simulink model "IM_DTC_controller_sim"  (R2023a)
settings: Solver=ode113  StartTime=0.0  StopTime=100.0  RelTol=1e-3
values from neighbouring files (symbols this model uses):
  B = 0.068    [IM_DTC_controller_param.m]
  DT = 0.001    [IM_DTC_controller_param.m]
  f = 50    [IM_DTC_controller_param.m]
  J = 0.4    [IM_DTC_controller_param.m]
  k = 0.009    [IM_DTC_controller_param.m]
  kiw = 0.068*1000    (= 68)    [IM_DTC_controller_param.m]
  kpw = 0.4*1000    (= 400)    [IM_DTC_controller_param.m]
  Lks = Ls- Lm^2/Lr    (= 0.00442538071066)    [IM_DTC_controller_param.m]
  Lm = 57e-3    (= 0.057)    [IM_DTC_controller_param.m]
  np = 3    [IM_DTC_controller_param.m]
  r = 4    [IM_DTC_controller_param.m]
  Rr = 0.175    [IM_DTC_controller_param.m]
  Rs = 0.24    [IM_DTC_controller_param.m]
  Rw = wc_des_w*(B+J*s)/s    [IM_DTC_controller_param.m]
  vsat = 380    [IM_DTC_controller_param.m]
  Ys_n = 1.71    [IM_DTC_controller_param.m]
undefined symbols (not defined in the file or in its folder): j
libraries: eeTransforms x5, sharedTrackingLibrary x1, slpidlib x1
settings Model: Creator=Andrea  LastModifiedBy=Andrea
settings SolverCC: ZeroCrossAlgorithm=Adaptive

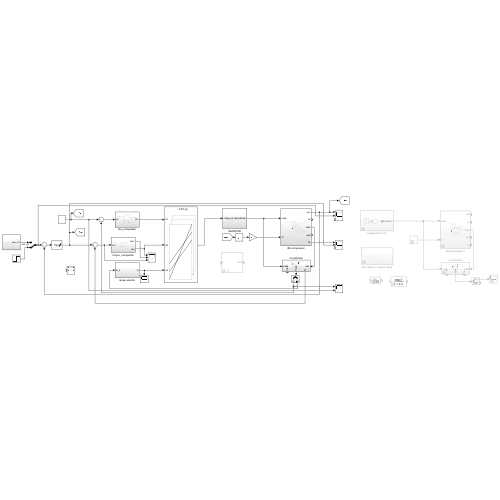
[thumbnail: Simulink's stored preview of the top-level diagram]
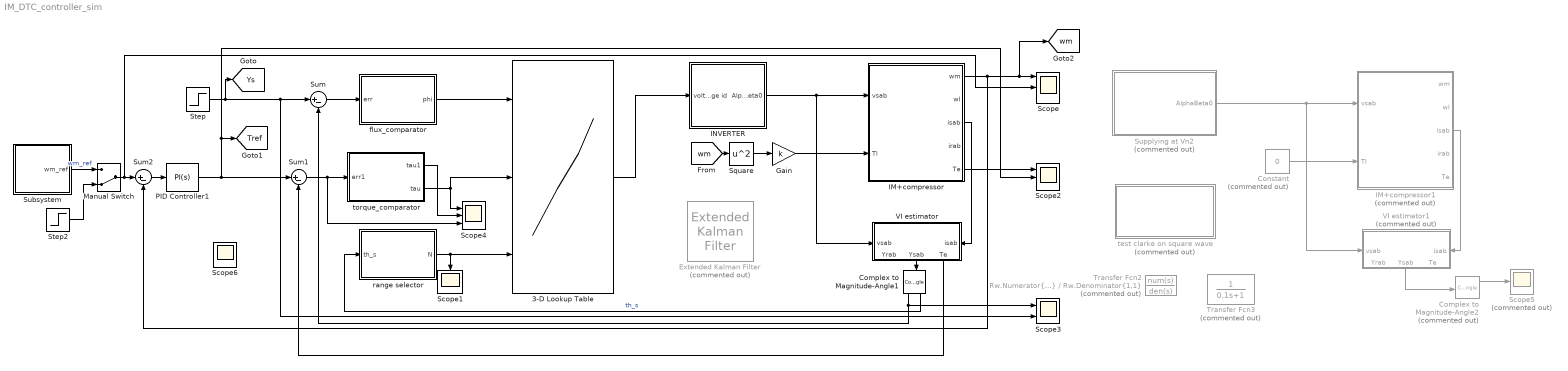
== system IM_DTC_controller_sim ==
  3-D Lookup Table : Lookup_n-D  NumberOfTableDimensions=3  BreakpointsForDimension1=[0;1]  BreakpointsForDimension2=[-1 0 1]  BreakpointsForDimension3=[1;2;3;4;5;6]  Table=reshape([1 5 0 7 2 6 5 4 7 0 3 2 4 6 0 7 1 3 6 2 7 0 5 1 2 3 0 7 4 5 3 1 7 0 6 4], [2 3 6])  InternalRulePriority=Speed  RndMeth=Simplest
      settings: InputPortMap=u0,u1,u2
  Complex to Magnitude-Angle1 : ComplexToMagnitudeAngle
  Complex to Magnitude-Angle2 : ComplexToMagnitudeAngle  Commented=on
  Constant : Constant  Commented=on  Value=0
  Extended Kalman Filter : sharedTrackingLibrary/Extended Kalman Filter  Commented=on  StateTransitionFcn=myStateTransitionFcn  HasStateTransitionJacobianFcn=off  HasAdditiveProcessNoise=Additive  ProcessNoise=1  HasTimeVaryingProcessNoise=off  HasStateTransitionFcnExtraArgument=0  InitialState=0  InitialStateCovariance=1  MeasurementFcn1=myMeasurementFcn  HasMeasurementJacobianFcn1=off  HasMeasurementEnablePort1=off  HasAdditiveMeasurementNoise1=Additive  MeasurementNoise1=1  HasTimeVaryingMeasurementNoise1=off  HasMeasurementFcnExtraArgument1=0  HasMeasurementWrapping1=off  MeasurementFcn2=myMeasurementFcn  HasMeasurementJacobianFcn2=off  HasMeasurementEnablePort2=off  HasAdditiveMeasurementNoise2=Additive  MeasurementNoise2=1  HasTimeVaryingMeasurementNoise2=off  HasMeasurementFcnExtraArgument2=0  HasMeasurementWrapping2=off  MeasurementFcn3=myMeasurementFcn  HasMeasurementJacobianFcn3=off  HasMeasurementEnablePort3=off  HasAdditiveMeasurementNoise3=Additive  MeasurementNoise3=1  HasTimeVaryingMeasurementNoise3=off  HasMeasurementFcnExtraArgument3=0  HasMeasurementWrapping3=off  MeasurementFcn4=myMeasurementFcn  HasMeasurementJacobianFcn4=off  HasMeasurementEnablePort4=off  HasAdditiveMeasurementNoise4=Additive  MeasurementNoise4=1  HasTimeVaryingMeasurementNoise4=off  HasMeasurementFcnExtraArgument4=0  HasMeasurementWrapping4=off  MeasurementFcn5=myMeasurementFcn  HasMeasurementJacobianFcn5=off  HasMeasurementEnablePort5=off  HasAdditiveMeasurementNoise5=Additive  MeasurementNoise5=1  HasTimeVaryingMeasurementNoise5=off  HasMeasurementFcnExtraArgument5=0  HasMeasurementWrapping5=off  EnableMultirate=off  StateTransitionFcnSampleTime=1  MeasurementFcn1SampleTime=1  MeasurementFcn2SampleTime=1  MeasurementFcn3SampleTime=1  MeasurementFcn4SampleTime=1  MeasurementFcn5SampleTime=1  UseCurrentEstimator=on  OutputStateCovariance=off  DataType=double  SampleTime=1  NumberOfMeasurements=1
  Gain : Gain  Gain=k
  IM+compressor : Subsystem
  IM+compressor1 : Subsystem  Commented=on
  INVERTER : Subsystem
  Manual Switch : ManualSwitch  CurrentSetting=0
  PID Controller1 : slpidlib/PID Controller  Controller=PI  Form=Parallel  TimeDomain=Continuous-time  UseExternalTs=off  SampleTime=-1  IntegratorMethod=Forward Euler  FilterMethod=Forward Euler  ControllerParametersSource=internal  P=kpw  I=kiw  UseKiTs=off  D=0  N=100  UseFilter=on  TunerSelectOption=Transfer Function Based (PID Tuner App)  InitialConditionSource=internal  InitialConditionForIntegrator=0  InitialConditionForFilter=0  DifferentiatorICPrevScaledInput=0  ExternalReset=none  TrackingMode=off  Kt=1  LimitOutput=on  SatLimitsSource=internal  UpperSaturationLimit=700  LowerSaturationLimit=-700  LinearizeAsGain=on  AntiWindupMode=back-calculation  Kb=kiw/kpw/5  LimitIntegrator=off  UpperIntegratorSaturationLimit=inf  LowerIntegratorSaturationLimit=-inf  POutMin=[]  POutMax=[]  IOutMin=[]  IOutMax=[]  DOutMin=[]  DOutMax=[]  NOutMin=[]  NOutMax=[]  SumOutMin=[]  SumOutMax=[]  SaturationOutMin=[]  SaturationOutMax=[]  PParamMin=[]  PParamMax=[]  IParamMin=[]  IParamMax=[]  DParamMin=[]  DParamMax=[]  NParamMin=[]  NParamMax=[]  KbParamMin=[]  KbParamMax=[]  KtParamMin=[]  KtParamMax=[]  KbOutMin=[]  KbOutMax=[]  KtOutMin=[]  KtOutMax=[]  IntegratorOutMin=[]  IntegratorOutMax=[]  FilterOutMin=[]  FilterOutMax=[]  SumI1OutMin=[]  SumI1OutMax=[]  SumI2OutMin=[]  SumI2OutMax=[]  SumI3OutMin=[]  SumI3OutMax=[]  SumI4OutMin=[]  SumI4OutMax=[]  SumDOutMin=[]  SumDOutMax=[]  DifferentiatorOutMin=[]  DifferentiatorOutMax=[]  FilterDiffOutCoefMin=[]  FilterDiffOutCoefMax=[]  ReciprocalOutMin=[]  ReciprocalOutMax=[]  SumDenOutMin=[]  SumDenOutMax=[]  SumNumOutMin=[]  SumNumOutMax=[]  DivideOutMin=[]  DivideOutMax=[]  UdiffTsProdOutMin=[]  UdiffTsProdOutMax=[]  NTsProdOutMin=[]  NTsProdOutMax=[]  UintegralTsProdOutMin=[]  UintegralTsProdOutMax=[]  UngainTsProdOutMin=[]  UngainTsProdOutMax=[]  ClampingZeroOutDataTypeStr=Inherit: Inherit via back propagation  ClampingZeroOutMin=[]  ClampingZeroOutMax=[]  FilterDenConstantOutDataTypeStr=Inherit: Inherit via back propagation  FilterDenConstantOutMin=[]  FilterDenConstantOutMax=[]  PCopyOutDataTypeStr=Inherit: Inherit via back propagation  PCopyOutMin=[]  PCopyOutMax=[]  NCopyOutDataTypeStr=Inherit: Inherit via back propagation  NCopyOutMin=[]  NCopyOutMax=[]  IntegratorContinuousStateAttributes=''  IntegratorStateMustResolveToSignalObject=off  IntegratorRTWStateStorageClass=Auto  FilterContinuousStateAttributes=''  FilterStateMustResolveToSignalObject=off  FilterRTWStateStorageClass=Auto  ParallelPVariant=InternalParameters  IdealPVariant=Disabled  IVariant=InternalParameters  DVariant=Disabled  IntegratorVariant=Continuous  SatVariant=Enabled  AWVariant=BackCalculation  PCopyVariant=Disabled  TRVariant=Disabled  FdbkBlocksVariant=Forward  IdealPFdbkVariant=Disabled  SatFdbkVariant=Disabled  DerivativeFilterVariant=Disabled  NVariant=Disabled  NCopyVariant=Disabled_SignalSpec  FilterICVariant=Disabled  IntegratorICVariant=InternalICs  ExternalResetVariant=Disabled  TRSumVariant=Passthrough  SumFdbkVariant=Disabled  SumVariant=Sum_PI  TsampFilterVariant=InternalTs  TsampNgainVariant=Passthrough  TsampIntegralVariant=Disabled_SignalSpec  ExternalSaturationOutDataTypeStr=Inherit: Same as second input
  Scope : Scope  NumInputPorts=3
  Scope1 : Scope
  Scope2 : Scope  NumInputPorts=3
  Scope3 : Scope  NumInputPorts=2
  Scope4 : Scope  NumInputPorts=3
  Scope5 : Scope  Commented=on
  Scope6 : Scope
  Square : Math  Operator=square
  Step : Step  Time=0  After=Ys_n  SampleTime=0
  Step2 : Step  After=50  SampleTime=0
  Subsystem : Subsystem
  Sum : Sum  Inputs=|+-
  Sum1 : Sum  Inputs=|+-
  Sum2 : Sum  Inputs=|+-
  Supplying at Vn2 : Subsystem  Commented=on
  Transfer Fcn2 : TransferFcn  Commented=on  Numerator=Rw.Numerator{1,1}  Denominator=Rw.Denominator{1,1}
  Transfer Fcn3 : TransferFcn  Commented=on  Denominator=[0.1 1]
  VI estimator : Subsystem
      settings: PortSchema="{\"entries\":[{\"content\":{\"sides\":[{\"content\":{},\"type\":\"ConnectorPlacement.EquallySpacedRectSide\",\"uuid\":\"e33eea5d-c803-4efd-b963-b28e7fd3b846\"},{\"content\":{\"connectorIds\":[\"Out1\",\"Out2\",\"Out3\"],\"side\":\"RIGHT\"},\"type\":\"ConnectorPlacement.EquallySpacedRectSide\",\"uuid\":\"16dd9f0c-f93f-4294-bb00-4f02950fe655\"},{\"content\":{\"connectorIds\":[\"In1\"],\"side\":\"TOP\"},\"type\":\"ConnectorPlacement.EquallySpacedRectSide\",\"uuid\":\"0c6e3d24-7610-41dc-8be5-eb5e396d3954\"},{\"content\":{\"connectorIds\":[\"In2\"],\"side\":\"BOTTOM\"},\"type\":\"ConnectorPlacement.EquallySpacedRectSide\",\"uuid\":\"785fd01a-f2d8-4593-9bc3-fce65e17d3d8\"}]},\"type\":\"ConnectorPlacement.EquallySpacedConnector\",\"uuid\":\"dc648cf4-6df6-4217-8a75-6fc5bc573b99\"}],\"packageUris\":[\"http://schema.mathworks.com/mf0/Connector/R2020b\"],\"version\":\"1.0\"}"
  VI estimator1 : Subsystem  Commented=on
      settings: PortSchema="{\"entries\":[{\"content\":{\"sides\":[{\"content\":{},\"type\":\"ConnectorPlacement.EquallySpacedRectSide\",\"uuid\":\"e33eea5d-c803-4efd-b963-b28e7fd3b846\"},{\"content\":{\"connectorIds\":[\"Out1\",\"Out2\",\"Out3\"],\"side\":\"RIGHT\"},\"type\":\"ConnectorPlacement.EquallySpacedRectSide\",\"uuid\":\"16dd9f0c-f93f-4294-bb00-4f02950fe655\"},{\"content\":{\"connectorIds\":[\"In1\"],\"side\":\"TOP\"},\"type\":\"ConnectorPlacement.EquallySpacedRectSide\",\"uuid\":\"0c6e3d24-7610-41dc-8be5-eb5e396d3954\"},{\"content\":{\"connectorIds\":[\"In2\"],\"side\":\"BOTTOM\"},\"type\":\"ConnectorPlacement.EquallySpacedRectSide\",\"uuid\":\"785fd01a-f2d8-4593-9bc3-fce65e17d3d8\"}]},\"type\":\"ConnectorPlacement.EquallySpacedConnector\",\"uuid\":\"dc648cf4-6df6-4217-8a75-6fc5bc573b99\"}],\"packageUris\":[\"http://schema.mathworks.com/mf0/Connector/R2020b\"],\"version\":\"1.0\"}"
  flux_comparator : Subsystem
  range selector : Subsystem
  test clarke on square wave : Subsystem  Commented=on
  torque_comparator : Subsystem
  tag scope: Tref=global, Ys=global, wm=global
  wires:
  Sum1/1 -> Scope4/3, torque_comparator/1(err1)
  Sum/1 -> flux_comparator/1(err)
  INVERTER/1(AlphaBeta0) -> VI estimator/2(vsab), IM+compressor/1(vsab)
  IM+compressor/3(isab) -> VI estimator/1(isab)
  VI estimator/2(Ysab) -> Complex to Magnitude-Angle1/1
  flux_comparator/1(phi) -> 3-D Lookup Table/1
  3-D Lookup Table/1 -> INVERTER/1(voltage id)
  Step/1 -> [Ys], Scope3/2, Sum/1
  IM+compressor/5(Te) -> Scope2/1
  Complex to Magnitude-Angle1/1 -> Sum/2, Scope3/1
  range selector/1(N) -> 3-D Lookup Table/3, Scope1/1
  Complex to Magnitude-Angle1/2 -> range selector/1(th_s)  "th_s"
  Sum2/1 -> PID Controller1/1
  Supplying at Vn2/1(AlphaBeta0) -> VI estimator1/2(vsab), IM+compressor1/1(vsab)
  IM+compressor1/3(isab) -> VI estimator1/1(isab)
  Constant/1 -> IM+compressor1/2(Tl)
  VI estimator1/2(Ysab) -> Complex to Magnitude-Angle2/1
  Step2/1 -> Manual Switch/2
  Complex to Magnitude-Angle2/1 -> Scope5/1
  torque_comparator/2(tau) -> 3-D Lookup Table/2, Scope4/1
  Manual Switch/1 -> Scope/2, Sum2/1
  Subsystem/1(wm_ref) -> Manual Switch/1  "wm_ref"
  PID Controller1/1 -> Sum1/1, Scope2/2, [Tref]
  VI estimator/1(Te) -> Sum1/2
  [wm] -> Square/1
  Gain/1 -> IM+compressor/2(Tl)
  Square/1 -> Gain/1
  IM+compressor/1(wm) -> Sum2/2, [wm], Scope/1
  torque_comparator/1(tau1) -> Scope4/2

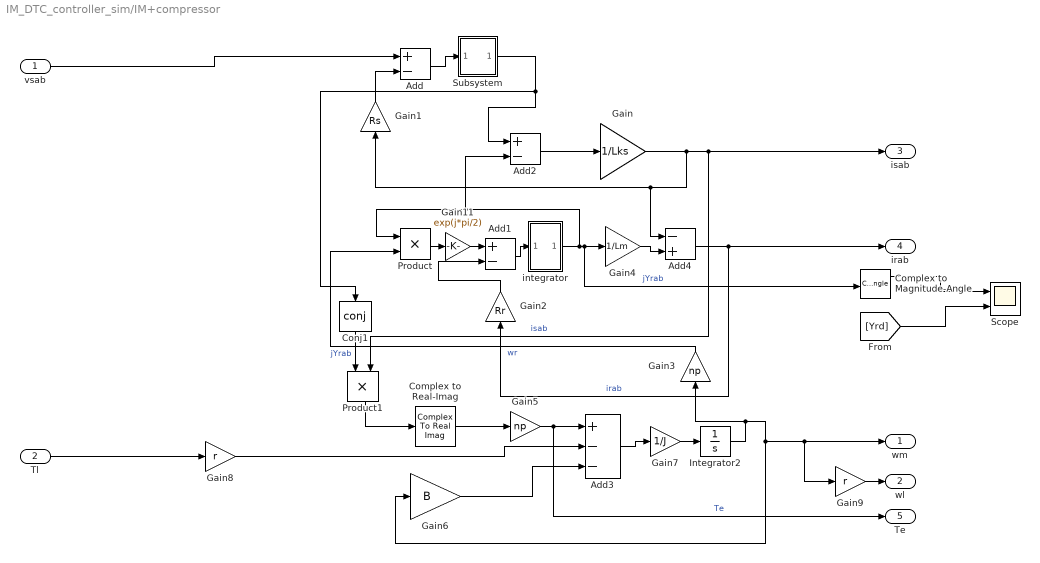
== system IM_DTC_controller_sim/IM+compressor ==
  vsab : Inport
  Tl : Inport  Port=2
  Add : Sum  Inputs=+-
  Add1 : Sum  Inputs=+-
  Add2 : Sum  Inputs=+-
  Add3 : Sum  Inputs=+--
  Add4 : Sum  Inputs=-+
  Complex to Magnitude-Angle : ComplexToMagnitudeAngle
  Complex to Real-Imag : ComplexToRealImag  Output=Imag
  Conj1 : Math  Operator=conj
  Gain : Gain  Gain=1/Lks
  Gain1 : Gain  Gain=Rs
  Gain11 : Gain  Gain=exp(j*pi/2)
  Gain2 : Gain  Gain=Rr
  Gain3 : Gain  Gain=np
  Gain4 : Gain  Gain=1/Lm
  Gain5 : Gain  Gain=np
  Gain6 : Gain  Gain=B
  Gain7 : Gain  Gain=1/J
  Gain8 : Gain  Gain=r
  Gain9 : Gain  Gain=r
  Integrator2 : Integrator
  Product : Product
  Product1 : Product
  Scope : Scope  NumInputPorts=2
  Subsystem : Subsystem
  integrator : Subsystem
  wm : Outport
  wl : Outport  Port=2
  isab : Outport  Port=3
      settings: SignalType=complex
  irab : Outport  Port=4
      settings: SignalType=complex
  Te : Outport  Port=5
  wires:
  Add2/1 -> Gain/1
  Add4/1 -> Gain2/1, irab/1  "irab"
  Gain/1 -> Add4/1, Gain1/1, Product1/2, isab/1  "isab"
  Gain6/1 -> Add3/3
  Gain4/1 -> Add4/2
  integrator/1(Yrab) -> Complex to Magnitude-Angle/1, Gain4/1, Product/1, Add2/2  "jYrab"
  Gain1/1 -> Add/2
  Gain5/1 -> Te/1, Add3/1  "Te"
  Product1/1 -> Complex to Real-Imag/1
  Conj1/1 -> Product1/1  "jYrab"
  Complex to Real-Imag/1 -> Gain5/1
  Gain2/1 -> Add1/2
  Add3/1 -> Gain7/1
  Gain7/1 -> Integrator2/1
  Gain3/1 -> Product/2  "wr"
  vsab/1 -> Add/1
  Tl/1 -> Gain8/1
  Add1/1 -> integrator/1(In1)
  Subsystem/1(Ysab) -> Add2/1, Conj1/1
  Add/1 -> Subsystem/1(In1)
  Gain11/1 -> Add1/1
  Product/1 -> Gain11/1
  Gain8/1 -> Add3/2
  Integrator2/1 -> Gain9/1, wm/1, Gain6/1, Gain3/1
  Gain9/1 -> wl/1
  [Yrd] -> Scope/2
  Complex to Magnitude-Angle/1 -> Scope/1

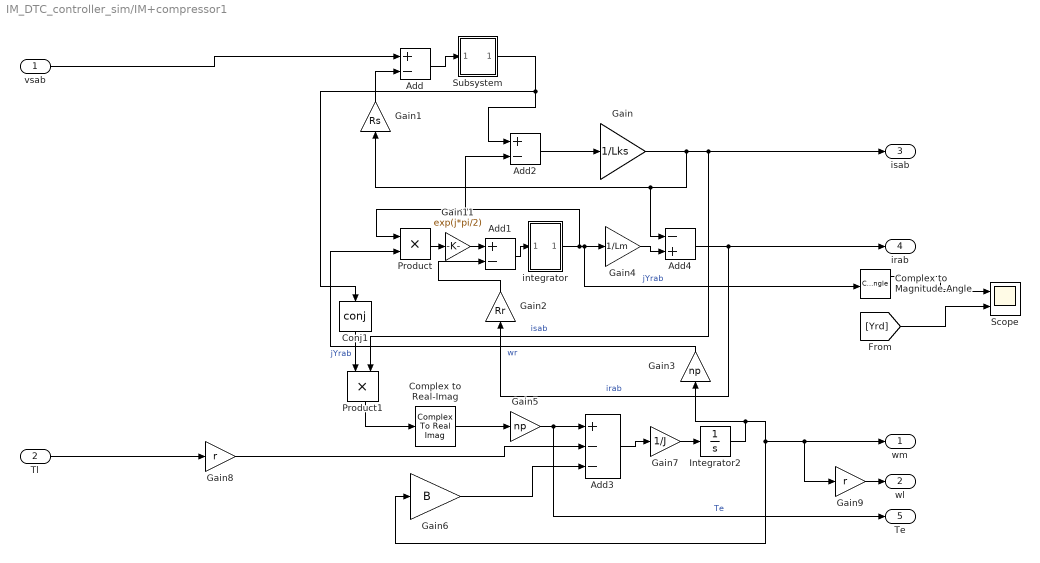
== system IM_DTC_controller_sim/IM+compressor1 ==
  vsab : Inport
  Tl : Inport  Port=2
  Add : Sum  Inputs=+-
  Add1 : Sum  Inputs=+-
  Add2 : Sum  Inputs=+-
  Add3 : Sum  Inputs=+--
  Add4 : Sum  Inputs=-+
  Complex to Magnitude-Angle : ComplexToMagnitudeAngle
  Complex to Real-Imag : ComplexToRealImag  Output=Imag
  Conj1 : Math  Operator=conj
  Gain : Gain  Gain=1/Lks
  Gain1 : Gain  Gain=Rs
  Gain11 : Gain  Gain=exp(j*pi/2)
  Gain2 : Gain  Gain=Rr
  Gain3 : Gain  Gain=np
  Gain4 : Gain  Gain=1/Lm
  Gain5 : Gain  Gain=np
  Gain6 : Gain  Gain=B
  Gain7 : Gain  Gain=1/J
  Gain8 : Gain  Gain=r
  Gain9 : Gain  Gain=r
  Integrator2 : Integrator
  Product : Product
  Product1 : Product
  Scope : Scope  NumInputPorts=2
  Subsystem : Subsystem
  integrator : Subsystem
  wm : Outport
  wl : Outport  Port=2
  isab : Outport  Port=3
      settings: SignalType=complex
  irab : Outport  Port=4
      settings: SignalType=complex
  Te : Outport  Port=5
  wires:
  Add2/1 -> Gain/1
  Add4/1 -> Gain2/1, irab/1  "irab"
  Gain/1 -> Add4/1, Gain1/1, Product1/2, isab/1  "isab"
  Gain6/1 -> Add3/3
  Gain4/1 -> Add4/2
  integrator/1(Yrab) -> Complex to Magnitude-Angle/1, Gain4/1, Product/1, Add2/2  "jYrab"
  Gain1/1 -> Add/2
  Gain5/1 -> Te/1, Add3/1  "Te"
  Product1/1 -> Complex to Real-Imag/1
  Conj1/1 -> Product1/1  "jYrab"
  Complex to Real-Imag/1 -> Gain5/1
  Gain2/1 -> Add1/2
  Add3/1 -> Gain7/1
  Gain7/1 -> Integrator2/1
  Gain3/1 -> Product/2  "wr"
  vsab/1 -> Add/1
  Tl/1 -> Gain8/1
  Add1/1 -> integrator/1(In1)
  Subsystem/1(Ysab) -> Add2/1, Conj1/1
  Add/1 -> Subsystem/1(In1)
  Gain11/1 -> Add1/1
  Product/1 -> Gain11/1
  Gain8/1 -> Add3/2
  Integrator2/1 -> Gain9/1, wm/1, Gain6/1, Gain3/1
  Gain9/1 -> wl/1
  [Yrd] -> Scope/2
  Complex to Magnitude-Angle/1 -> Scope/1

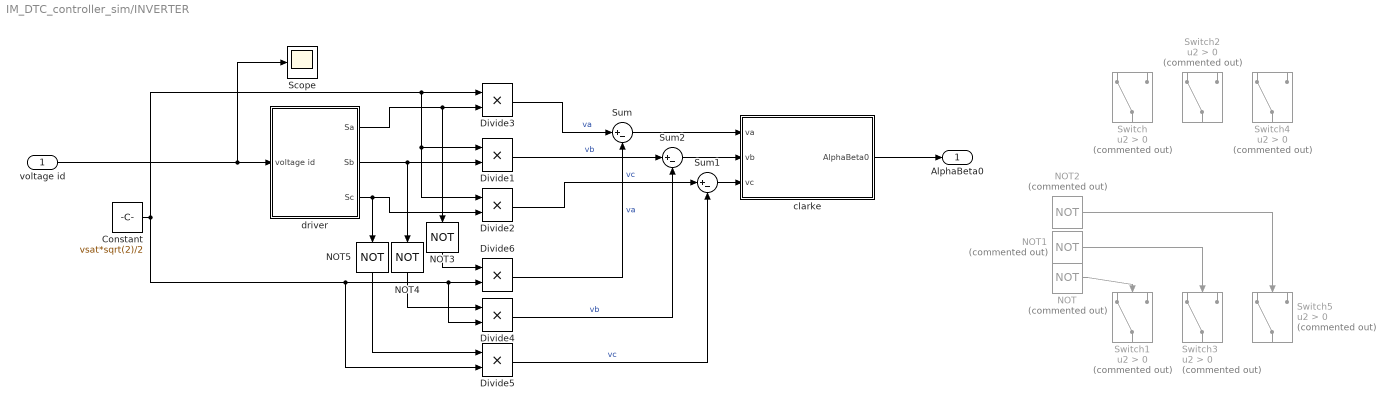
== system IM_DTC_controller_sim/INVERTER ==
  voltage id : Inport
  Constant : Constant  Value=vsat*sqrt(2)/2
  Divide{1..6} (6 alike) : Product  Inputs=**
  NOT : Logic  Commented=on  Operator=NOT  IconShape=distinctive  AllPortsSameDT=off  OutDataTypeStr=boolean
  NOT1 : Logic  Commented=on  Operator=NOT  IconShape=distinctive  AllPortsSameDT=off  OutDataTypeStr=boolean
  NOT2 : Logic  Commented=on  Operator=NOT  IconShape=distinctive  AllPortsSameDT=off  OutDataTypeStr=boolean
  NOT3 : Logic  Operator=NOT  IconShape=distinctive  AllPortsSameDT=off  OutDataTypeStr=boolean
  NOT4 : Logic  Operator=NOT  IconShape=distinctive  AllPortsSameDT=off  OutDataTypeStr=boolean
  NOT5 : Logic  Operator=NOT  IconShape=distinctive  AllPortsSameDT=off  OutDataTypeStr=boolean
  Scope : Scope
  Sum : Sum  Inputs=|+-
  Sum1 : Sum  Inputs=|+-
  Sum2 : Sum  Inputs=|+-
  Switch{,1..5} (6 alike) : Switch  Commented=on  Criteria=u2 > Threshold  SaturateOnIntegerOverflow=off  InputSameDT=off
  clarke : Subsystem
  driver : Subsystem
  AlphaBeta0 : Outport
  wires:
  voltage id/1 -> Scope/1, driver/1(voltage id)
  ? -> NOT/1, Switch/2
  ? -> Switch2/2, NOT1/1
  ? -> NOT2/1, Switch4/2
  NOT/1 -> Switch1/2
  NOT2/1 -> Switch5/2
  NOT1/1 -> Switch3/2
  driver/1(Sa) -> Divide3/2, NOT3/1
  driver/2(Sb) -> NOT4/1, Divide1/2
  driver/3(Sc) -> NOT5/1, Divide2/2
  clarke/1(AlphaBeta0) -> AlphaBeta0/1
  Divide3/1 -> Sum/1  "va"
  Divide2/1 -> Sum1/1  "vc"
  Divide1/1 -> Sum2/1  "vb"
  Sum2/1 -> clarke/2(vb)
  Sum/1 -> clarke/1(va)
  Sum1/1 -> clarke/3(vc)
  NOT3/1 -> Divide6/1
  NOT4/1 -> Divide4/1
  NOT5/1 -> Divide5/1
  Constant/1 -> Divide5/2, Divide4/2, Divide6/2, Divide2/1, Divide1/1, Divide3/1
  Divide6/1 -> Sum/2  "va"
  Divide4/1 -> Sum2/2  "vb"
  Divide5/1 -> Sum1/2  "vc"

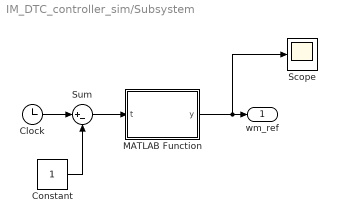
== system IM_DTC_controller_sim/Subsystem ==
  Clock : Clock
  Constant : Constant
  MATLAB Function : MATLAB Function  TreatAsAtomicUnit=on
  Scope : Scope
  Sum : Sum  Inputs=|+-
  wm_ref : Outport
  wires:
  MATLAB Function/1(y) -> Scope/1, wm_ref/1
  Clock/1 -> Sum/1
  Sum/1 -> MATLAB Function/1(t)
  Constant/1 -> Sum/2

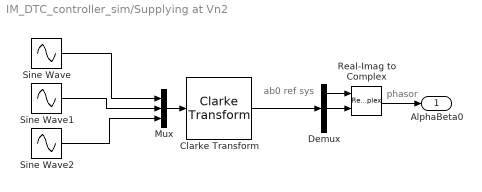
== system IM_DTC_controller_sim/Supplying at Vn2 ==
  note: ab0 ref sys
  note: phasor
  Clarke Transform : eeTransforms/Clarke Transform  PowerInvariant=off
      settings: LibrarySourceBlock=|
      | ee_sl_lib/Mathematical
      | Transforms/Clarke Transform
  Demux : Demux  Outputs=3
  Mux : Mux  Inputs=3
  Real-Imag to Complex : RealImagToComplex
  Sine Wave : Sin  Amplitude=vsat*sqrt(2)  Frequency=f*2*pi  SampleTime=0
  Sine Wave1 : Sin  Amplitude=vsat*sqrt(2)  Frequency=f*2*pi  Phase=-2/3*pi  SampleTime=0
  Sine Wave2 : Sin  Amplitude=vsat*sqrt(2)  Frequency=f*2*pi  Phase=-4/3*pi  SampleTime=0
  AlphaBeta0 : Outport
  wires:
  Real-Imag to Complex/1 -> AlphaBeta0/1
  Demux/1 -> Real-Imag to Complex/1
  Clarke Transform/1 -> Demux/1
  Demux/2 -> Real-Imag to Complex/2
  Sine Wave1/1 -> Mux/2
  Sine Wave2/1 -> Mux/3
  Mux/1 -> Clarke Transform/1
  Sine Wave/1 -> Mux/1

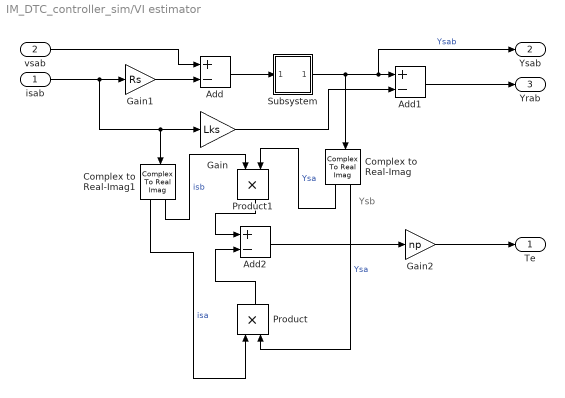
== system IM_DTC_controller_sim/VI estimator ==
  note: Ysb
  isab : Inport
  vsab : Inport  Port=2
  Add : Sum  Inputs=+-
  Add1 : Sum  Inputs=+-
  Add2 : Sum  Inputs=+-
  Complex to Real-Imag : ComplexToRealImag
  Complex to Real-Imag1 : ComplexToRealImag
  Gain : Gain  Gain=Lks
  Gain1 : Gain  Gain=Rs
  Gain2 : Gain  Gain=np
  Product : Product
  Product1 : Product
  Subsystem : Subsystem
  Te : Outport
  Ysab : Outport  Port=2
  Yrab : Outport  Port=3
  wires:
  Subsystem/1(Ysab) -> Complex to Real-Imag/1, Ysab/1, Add1/1  "Ysab"
  Add/1 -> Subsystem/1(In1)
  Add1/1 -> Yrab/1
  vsab/1 -> Add/1
  Gain1/1 -> Add/2
  Gain/1 -> Add1/2
  isab/1 -> Complex to Real-Imag1/1, Gain/1, Gain1/1
  Complex to Real-Imag/1 -> Product1/2  "Ysa"
  Complex to Real-Imag/2 -> Product/2  "Ysa"
  Complex to Real-Imag1/1 -> Product/1  "isa"
  Product1/1 -> Add2/1
  Product/1 -> Add2/2
  Add2/1 -> Gain2/1
  Gain2/1 -> Te/1
  Complex to Real-Imag1/2 -> Product1/1  "isb"

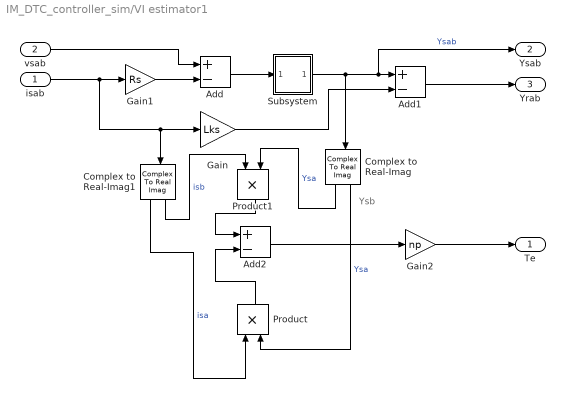
== system IM_DTC_controller_sim/VI estimator1 ==
  note: Ysb
  isab : Inport
  vsab : Inport  Port=2
  Add : Sum  Inputs=+-
  Add1 : Sum  Inputs=+-
  Add2 : Sum  Inputs=+-
  Complex to Real-Imag : ComplexToRealImag
  Complex to Real-Imag1 : ComplexToRealImag
  Gain : Gain  Gain=Lks
  Gain1 : Gain  Gain=Rs
  Gain2 : Gain  Gain=np
  Product : Product
  Product1 : Product
  Subsystem : Subsystem
  Te : Outport
  Ysab : Outport  Port=2
  Yrab : Outport  Port=3
  wires:
  Subsystem/1(Ysab) -> Complex to Real-Imag/1, Ysab/1, Add1/1  "Ysab"
  Add/1 -> Subsystem/1(In1)
  Add1/1 -> Yrab/1
  vsab/1 -> Add/1
  Gain1/1 -> Add/2
  Gain/1 -> Add1/2
  isab/1 -> Complex to Real-Imag1/1, Gain/1, Gain1/1
  Complex to Real-Imag/1 -> Product1/2  "Ysa"
  Complex to Real-Imag/2 -> Product/2  "Ysa"
  Complex to Real-Imag1/1 -> Product/1  "isa"
  Product1/1 -> Add2/1
  Product/1 -> Add2/2
  Add2/1 -> Gain2/1
  Gain2/1 -> Te/1
  Complex to Real-Imag1/2 -> Product1/1  "isb"

== system IM_DTC_controller_sim/flux_comparator ==
  err : Inport
  Memory : Memory
  flux comparator : MATLAB Function  TreatAsAtomicUnit=on
  phi : Outport
  wires:
  flux comparator/1(phi) -> phi/1, Memory/1
  err/1 -> flux comparator/1(err)
  Memory/1 -> flux comparator/2(old_phi)

== system IM_DTC_controller_sim/range selector ==
  th_s : Inport
  MATLAB Function : MATLAB Function  TreatAsAtomicUnit=on
  N : Outport
  wires:
  MATLAB Function/1(N) -> N/1
  th_s/1 -> MATLAB Function/1(th_s)

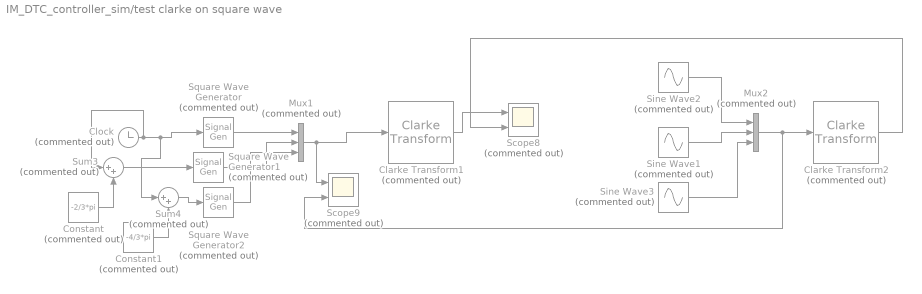
== system IM_DTC_controller_sim/test clarke on square wave ==
  Clarke Transform1 : eeTransforms/Clarke Transform  Commented=on  PowerInvariant=on
      settings: LibrarySourceBlock=|
      | ee_sl_lib/Mathematical
      | Transforms/Clarke Transform
  Clarke Transform2 : eeTransforms/Clarke Transform  Commented=on  PowerInvariant=on
      settings: LibrarySourceBlock=|
      | ee_sl_lib/Mathematical
      | Transforms/Clarke Transform
  Clock : Clock  Commented=on
  Constant : Constant  Commented=on  Value=-2/3*pi
  Constant1 : Constant  Commented=on  Value=-4/3*pi
  Mux1 : Mux  Commented=on  Inputs=3
  Mux2 : Mux  Commented=on  Inputs=3
  Scope8 : Scope  Commented=on  NumInputPorts=2
  Scope9 : Scope  Commented=on  NumInputPorts=2
  Sine Wave1 : Sin  Commented=on  Amplitude=380  Phase=-2/3*pi  SampleTime=0
  Sine Wave2 : Sin  Commented=on  Amplitude=380  SampleTime=0
  Sine Wave3 : Sin  Commented=on  Amplitude=380  Phase=-4/3*pi  SampleTime=0
  Square Wave Generator : SignalGenerator  Commented=on  WaveForm=square  TimeSource=Use external signal  Amplitude=-380  Units=rad/sec
  Square Wave Generator1 : SignalGenerator  Commented=on  WaveForm=square  TimeSource=Use external signal  Amplitude=-380  Units=rad/sec
  Square Wave Generator2 : SignalGenerator  Commented=on  WaveForm=square  TimeSource=Use external signal  Amplitude=-380  Units=rad/sec
  Sum3 : Sum  Commented=on  Inputs=|++
  Sum4 : Sum  Commented=on  Inputs=|++
  wires:
  Clock/1 -> Sum4/1, Square Wave Generator/1, Sum3/1
  Sum3/1 -> Square Wave Generator1/1
  Mux1/1 -> Scope9/1, Clarke Transform1/1
  Sine Wave2/1 -> Mux2/1
  Clarke Transform1/1 -> Scope8/1
  Constant/1 -> Sum3/2
  Sine Wave3/1 -> Mux2/3
  Sine Wave1/1 -> Mux2/2
  Square Wave Generator1/1 -> Mux1/2
  Square Wave Generator2/1 -> Mux1/3
  Mux2/1 -> Clarke Transform2/1, Scope9/2
  Clarke Transform2/1 -> Scope8/2
  Constant1/1 -> Sum4/2
  Sum4/1 -> Square Wave Generator2/1
  Square Wave Generator/1 -> Mux1/1

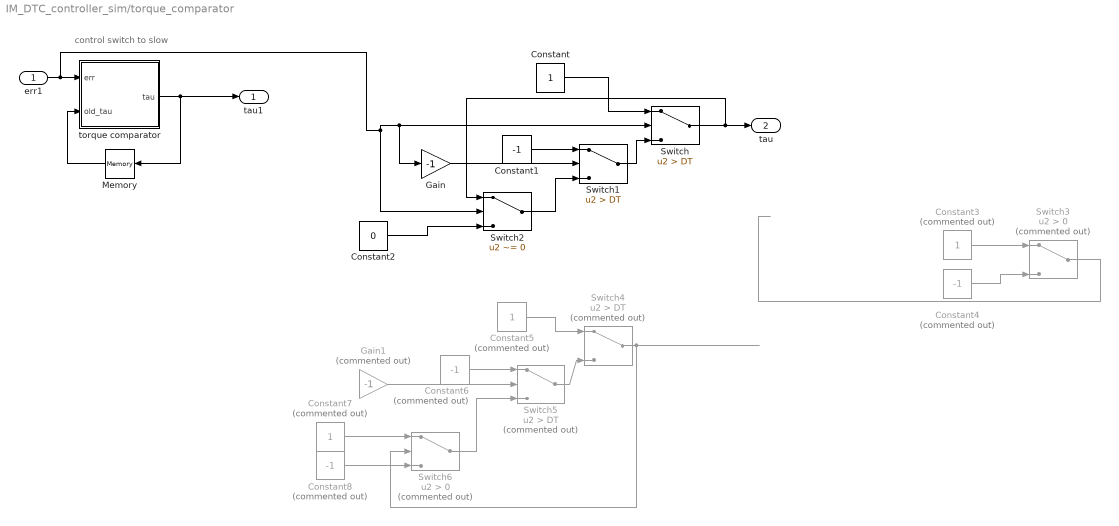
== system IM_DTC_controller_sim/torque_comparator ==
  note: control switch to slow
  err1 : Inport
  Constant : Constant
  Constant1 : Constant  Value=-1
  Constant2 : Constant  Value=0
  Constant3 : Constant  Commented=on
  Constant4 : Constant  Commented=on  Value=-1
  Constant5 : Constant  Commented=on
  Constant6 : Constant  Commented=on  Value=-1
  Constant7 : Constant  Commented=on
  Constant8 : Constant  Commented=on  Value=-1
  Gain : Gain  Gain=-1
  Gain1 : Gain  Commented=on  Gain=-1
  Memory : Memory  InheritSampleTime=on  LinearizeMemory=on  LinearizeAsDelay=on
  Switch : Switch  Criteria=u2 > Threshold  Threshold=DT  ZeroCross=off  SaturateOnIntegerOverflow=off  InputSameDT=off
  Switch1 : Switch  Criteria=u2 > Threshold  Threshold=DT  ZeroCross=off  SaturateOnIntegerOverflow=off  InputSameDT=off
  Switch2 : Switch  Criteria=u2 ~= 0  ZeroCross=off  SaturateOnIntegerOverflow=off  InputSameDT=off
  Switch3 : Switch  Commented=on  Criteria=u2 > Threshold  SaturateOnIntegerOverflow=off  InputSameDT=off
  Switch4 : Switch  Commented=on  Criteria=u2 > Threshold  Threshold=DT  SaturateOnIntegerOverflow=off  InputSameDT=off
  Switch5 : Switch  Commented=on  Criteria=u2 > Threshold  Threshold=DT  SaturateOnIntegerOverflow=off  InputSameDT=off
  Switch6 : Switch  Commented=on  Criteria=u2 > Threshold  SaturateOnIntegerOverflow=off  InputSameDT=off
  torque comparator : MATLAB Function  TreatAsAtomicUnit=on
  tau1 : Outport
  tau : Outport  Port=2
  wires:
  Memory/1 -> torque comparator/2(old_tau)
  torque comparator/1(tau) -> tau1/1, Memory/1
  Constant/1 -> Switch/1
  Switch1/1 -> Switch/3
  Constant1/1 -> Switch1/1
  err1/1 -> Gain/1, Switch/2, Switch2/2, torque comparator/1(err)
  Gain/1 -> Switch1/2
  Switch2/1 -> Switch1/3
  Constant2/1 -> Switch2/3
  Switch/1 -> tau/1, Switch2/1
  Constant5/1 -> Switch4/1
  Constant6/1 -> Switch5/1
  Switch6/1 -> Switch5/3
  ? -> Gain1/1, Switch4/2
  Gain1/1 -> Switch5/2
  Switch5/1 -> Switch4/3
  Constant8/1 -> Switch6/3
  Constant7/1 -> Switch6/1
  Switch4/1 -> Switch6/2
  Constant4/1 -> Switch3/3
  Switch3/1 -> ?
  Constant3/1 -> Switch3/1
  ? -> Switch3/2

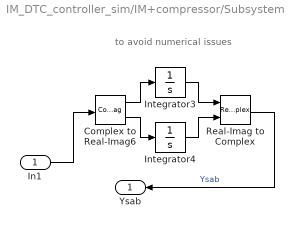
== system IM_DTC_controller_sim/IM+compressor/Subsystem ==
  note: to avoid numerical issues
  In1 : Inport
  Complex to Real-Imag6 : ComplexToRealImag
  Integrator3 : Integrator
  Integrator4 : Integrator
  Real-Imag to Complex : RealImagToComplex
  Ysab : Outport
  wires:
  In1/1 -> Complex to Real-Imag6/1
  Complex to Real-Imag6/2 -> Integrator4/1
  Complex to Real-Imag6/1 -> Integrator3/1
  Integrator3/1 -> Real-Imag to Complex/1
  Real-Imag to Complex/1 -> Ysab/1  "Ysab"
  Integrator4/1 -> Real-Imag to Complex/2

== system IM_DTC_controller_sim/IM+compressor/integrator ==
  In1 : Inport
  Complex to Real-Imag7 : ComplexToRealImag
  Integrator1 : Integrator
  Integrator5 : Integrator
  Real-Imag to Complex1 : RealImagToComplex
  Yrab : Outport
  wires:
  Complex to Real-Imag7/2 -> Integrator5/1
  Integrator1/1 -> Real-Imag to Complex1/1
  Real-Imag to Complex1/1 -> Yrab/1  "Yrab"
  Integrator5/1 -> Real-Imag to Complex1/2
  Complex to Real-Imag7/1 -> Integrator1/1
  In1/1 -> Complex to Real-Imag7/1

== system IM_DTC_controller_sim/IM+compressor1/Subsystem ==
  note: to avoid numerical issues
  In1 : Inport
  Complex to Real-Imag6 : ComplexToRealImag
  Integrator3 : Integrator
  Integrator4 : Integrator
  Real-Imag to Complex : RealImagToComplex
  Ysab : Outport
  wires:
  In1/1 -> Complex to Real-Imag6/1
  Complex to Real-Imag6/2 -> Integrator4/1
  Complex to Real-Imag6/1 -> Integrator3/1
  Integrator3/1 -> Real-Imag to Complex/1
  Real-Imag to Complex/1 -> Ysab/1  "Ysab"
  Integrator4/1 -> Real-Imag to Complex/2

== system IM_DTC_controller_sim/IM+compressor1/integrator ==
  In1 : Inport
  Complex to Real-Imag7 : ComplexToRealImag
  Integrator1 : Integrator
  Integrator5 : Integrator
  Real-Imag to Complex1 : RealImagToComplex
  Yrab : Outport
  wires:
  Complex to Real-Imag7/2 -> Integrator5/1
  Integrator1/1 -> Real-Imag to Complex1/1
  Real-Imag to Complex1/1 -> Yrab/1  "Yrab"
  Integrator5/1 -> Real-Imag to Complex1/2
  Complex to Real-Imag7/1 -> Integrator1/1
  In1/1 -> Complex to Real-Imag7/1

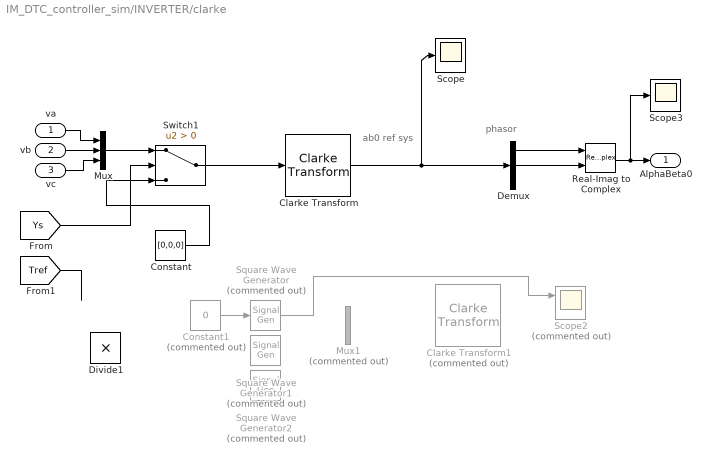
== system IM_DTC_controller_sim/INVERTER/clarke ==
  note: phasor
  note: ab0 ref sys
  va : Inport
  vb : Inport  Port=2
  vc : Inport  Port=3
  Clarke Transform : eeTransforms/Clarke Transform  PowerInvariant=on
      settings: LibrarySourceBlock=|
      | ee_sl_lib/Mathematical
      | Transforms/Clarke Transform
  Clarke Transform1 : eeTransforms/Clarke Transform  Commented=on  PowerInvariant=on
      settings: LibrarySourceBlock=|
      | ee_sl_lib/Mathematical
      | Transforms/Clarke Transform
  Constant : Constant  Value=[0,0,0]
  Constant1 : Constant  Commented=on  Value=0
  Demux : Demux  Outputs=3
  Divide1 : Product  Inputs=**
  Mux : Mux  Inputs=3
  Mux1 : Mux  Commented=on  Inputs=3
  Real-Imag to Complex : RealImagToComplex
  Scope : Scope
  Scope2 : Scope  Commented=on  NumInputPorts=2
  Scope3 : Scope
  Square Wave Generator : SignalGenerator  Commented=on  WaveForm=square  TimeSource=Use external signal  Amplitude=380  Units=rad/sec
  Square Wave Generator1 : SignalGenerator  Commented=on  WaveForm=square  Amplitude=380  Frequency=50*2*pi  Units=rad/sec
  Square Wave Generator2 : SignalGenerator  Commented=on  WaveForm=square  Amplitude=380  Frequency=50*2*pi  Units=rad/sec
  Switch1 : Switch  Criteria=u2 > Threshold  ZeroCross=off  SaturateOnIntegerOverflow=off  InputSameDT=off
  AlphaBeta0 : Outport
  wires:
  Demux/2 -> Real-Imag to Complex/2
  Demux/1 -> Real-Imag to Complex/1
  Real-Imag to Complex/1 -> Scope3/1, AlphaBeta0/1
  va/1 -> Mux/1
  vb/1 -> Mux/2
  vc/1 -> Mux/3
  Clarke Transform/1 -> Scope/1, Demux/1
  [Ys] -> Switch1/2
  [Tref] -> ?
  Constant/1 -> Switch1/3
  Mux/1 -> Switch1/1
  Square Wave Generator/1 -> Scope2/1
  Constant1/1 -> Square Wave Generator/1
  Switch1/1 -> Clarke Transform/1

== system IM_DTC_controller_sim/INVERTER/driver ==
  voltage id : Inport
  MATLAB Function : MATLAB Function  TreatAsAtomicUnit=on
  Scope : Scope
  Sa : Outport
  Sb : Outport  Port=2
  Sc : Outport  Port=3
  wires:
  voltage id/1 -> Scope/1, MATLAB Function/1(volt_id)
  MATLAB Function/1(Sa) -> Sa/1
  MATLAB Function/2(Sb) -> Sb/1
  MATLAB Function/3(Sc) -> Sc/1

== system IM_DTC_controller_sim/VI estimator/Subsystem ==
  note: to avoid numerical issues
  In1 : Inport
  Complex to Real-Imag6 : ComplexToRealImag
  Integrator3 : Integrator
  Integrator4 : Integrator
  Real-Imag to Complex : RealImagToComplex
  Ysab : Outport
  wires:
  In1/1 -> Complex to Real-Imag6/1
  Complex to Real-Imag6/2 -> Integrator4/1
  Complex to Real-Imag6/1 -> Integrator3/1
  Integrator3/1 -> Real-Imag to Complex/1
  Real-Imag to Complex/1 -> Ysab/1  "Ysab"
  Integrator4/1 -> Real-Imag to Complex/2

== system IM_DTC_controller_sim/VI estimator1/Subsystem ==
  note: to avoid numerical issues
  In1 : Inport
  Complex to Real-Imag6 : ComplexToRealImag
  Integrator3 : Integrator
  Integrator4 : Integrator
  Real-Imag to Complex : RealImagToComplex
  Ysab : Outport
  wires:
  In1/1 -> Complex to Real-Imag6/1
  Complex to Real-Imag6/2 -> Integrator4/1
  Complex to Real-Imag6/1 -> Integrator3/1
  Integrator3/1 -> Real-Imag to Complex/1
  Real-Imag to Complex/1 -> Ysab/1  "Ysab"
  Integrator4/1 -> Real-Imag to Complex/2

== matlab function IM_DTC_controller_sim/flux_comparator/flux comparator ==
  data: err input; phi output; old_phi input
function phi = fcn(err, old_phi)
DYs = .001;
if err <= -DYs
    phi = 0;
elseif err >= DYs
    phi = 1;
elseif err > -DYs && err < DYs
    phi = old_phi;
else 
    phi = 0;
end

== matlab function IM_DTC_controller_sim/range selector/MATLAB Function ==
  data: th_s input; N output
function N = fcn(th_s)
if th_s < pi/6 && th_s >= -pi/6
    N = 1;
elseif th_s > pi/6 && th_s <= pi/2
    N = 2;
elseif th_s > pi/2 && th_s <= 5/6*pi
    N = 3;
elseif (th_s > 5/6*pi && th_s < pi) || (th_s <= -5/6*pi && th_s >= -pi)
    N = 4;
elseif th_s > -5/6*pi && th_s <= -1/2*pi
    N = 5;
elseif th_s > -1/2*pi && th_s <= -1/6*pi
    N = 6;
else 
    N = 0;
end

== matlab function IM_DTC_controller_sim/INVERTER/driver/MATLAB Function ==
  data: volt_id input; Sa output; Sb output; Sc output
function [Sa,Sb,Sc] = fcn(volt_id)
    if volt_id == 0
        Sa = 0;
        Sb = 0;
        Sc = 0;
    elseif volt_id == 1
        Sa = 0;
        Sb = 0;
        Sc = 1;
    elseif volt_id == 2
        Sa = 0;
        Sb = 1;
        Sc = 0;
    elseif volt_id == 3
        Sa = 0;
        Sb = 1;
        Sc = 1;
    elseif volt_id == 4
        Sa = 1;
        Sb = 0;
        Sc = 0;
    elseif volt_id == 5
        Sa = 1;
        Sb = 0;
        Sc = 1;
    elseif volt_id == 6
        Sa = 1;
        Sb = 1;
        Sc = 0;
    elseif volt_id == 7
        Sa = 1;
        Sb = 1;
        Sc = 1;
    else 
        Sa = 0;
        Sb = 0;
        Sc = 0;
    end

== matlab function IM_DTC_controller_sim/Subsystem/MATLAB Function ==
  data: t input; y output
function y = fcn(t)
wm_n = 104.6;
if t<=0
    y = 0;
elseif t<20 && t>0
    y = t*0.005*wm_n; 
elseif t>=20 && t<30
    y = 0.1*wm_n;
elseif t>=30 && t<40
    y = t*0.01*wm_n-0.2*wm_n;
else
    y = 0.2*wm_n;
end

== matlab function IM_DTC_controller_sim/torque_comparator/torque comparator ==
  data: err input; tau output; old_tau input
function tau = fcn(err, old_tau)
DT = .01;
if err > 0
    if err >= DT
        tau = 1;
    else
        % if old_tau == -1
        %     tau = -old_tau;
        % else 
            tau = old_tau;
        % end
    end
elseif err < 0
    if err <= -DT
        tau = -1;
    else
        % if old_tau == 1
        %     tau = -old_tau;
        % else 
            tau = old_tau;
        % end
    end
else 
    tau = 0;
end
